simulink model "SMR_1MW_model"  (R2025b)
settings: Solver=daessc  StartTime=0.0  StopTime=60*80  RelTol=1e-3
libraries: fl_lib x41, nesl_utility x29, RankineCycle_lib x3, simulink x2, slpidlib x2
(part 2 of 2)

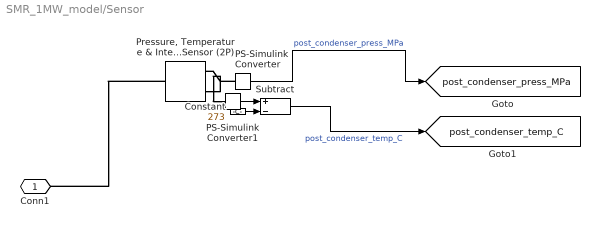
== system SMR_1MW_model/Sensor ==
  Constant : Constant  Value=273
  PS-Simulink Converter : nesl_utility/PS-Simulink Converter  PhysicalDomain=network_engine_domain  SubClassName=ps_output  LeftPortType=input  RightPortType=output  PseudoPeriodic=off  Frequencies=[]  VectorFormat=inherit  Unit=inherit  AffineConversion=off
  PS-Simulink Converter1 : nesl_utility/PS-Simulink Converter  PhysicalDomain=network_engine_domain  SubClassName=ps_output  LeftPortType=input  RightPortType=output  PseudoPeriodic=off  Frequencies=[]  VectorFormat=inherit  Unit=inherit  AffineConversion=off
  "Pressure, Temperature & Internal Energy Sensor (2P)" : fl_lib/Two-Phase Fluid/Sensors/Pressure, Temperature & Internal Energy Sensor (2P)  reference=foundation.enum.MeasurementReference.absolute  pressure=true  pressure_spec=foundation.enum.PressureMeasementSpec.Absolute  temperature=true  internal_energy=false
      settings: InternalSimscapePortConfiguration="{\"Bottom\":[{\"id\":\"T\",\"label\":\"T\",\"type\":\"output\"}],\"Left\":[{\"id\":\"A\",\"label\":\"A\",\"type\":\"foundation.two_phase_fluid.two_phase_fluid\"}],\"Right\":[{\"id\":\"Pa\",\"label\":\"Pa\",\"type\":\"output\"}],\"Top\":[]}"
  Subtract : Sum  Inputs=+-
  Conn1 : PMIOPort  Side=Left
  tag scope: post_condenser_press_MPa=global, post_condenser_temp_C=global
  wires:
  PS-Simulink Converter/1 -> [post_condenser_press_MPa]  "post_condenser_press_MPa"
  PS-Simulink Converter1/1 -> Subtract/1
  Constant/1 -> Subtract/2
  Subtract/1 -> [post_condenser_temp_C]  "post_condenser_temp_C"
  connections:
  PS-Simulink Converter/LConn1 -- "Pressure, Temperature & Internal Energy Sensor (2P)"/RConn1
  "Pressure, Temperature & Internal Energy Sensor (2P)"/RConn2 -- PS-Simulink Converter1/LConn1
  "Pressure, Temperature & Internal Energy Sensor (2P)"/LConn1 -- Conn1/RConn1

== system SMR_1MW_model/Sensors ==
  Subsystem4 : Subsystem
  Conn1 : PMIOPort  Side=Right
  tag scope: pre_trubine_temp_C=global, pre_turbine_press_MPa=global
  wires:
  Subsystem4/1(pressure) -> [pre_turbine_press_MPa]  "pre-turbine_press_MPa"
  Subsystem4/2(temperature) -> [pre_trubine_temp_C]  "pre-trubine_temp_C"
  connections:
  Subsystem4/LConn1 -- Conn1/RConn1

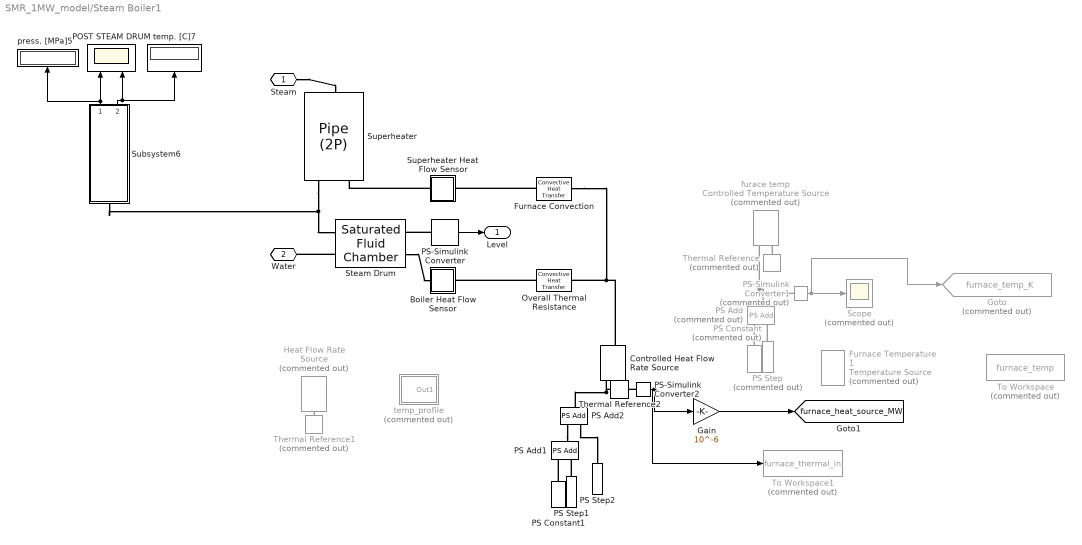
== system SMR_1MW_model/Steam Boiler1 ==
  Boiler Heat Flow Sensor : Subsystem
  Controlled Heat Flow Rate Source : fl_lib/Thermal/Thermal Sources/Controlled Heat Flow Rate Source
  Furnace Convection : fl_lib/Thermal/Thermal Elements/Convective Heat Transfer  thermal_type=foundation.enum.constant_variable.constant  area=pi * sqrt(4*0.01/pi) * 4+ 2 m^2  heat_tr_coeff=heater_heat_coeff W/(m^2 * K)  min_heat_tr_coeff=1e-3 W/(K*m^2)  T_specify=off  T_priority=None  T=0 K  T_nominal_specify=off  T_nominal_value=1  T_nominal_unit=K  Q_specify=off  Q_priority=None  Q=0 W  Q_nominal_specify=off  Q_nominal_value=1  Q_nominal_unit=W
  Furnace Temperature1 : fl_lib/Thermal/Thermal Sources/Temperature Source  Commented=on  temperature=T_furnace degC
  Gain : Gain  Gain=10^-6
  Goto : Goto  Commented=on  GotoTag=furnace_temp_K  TagVisibility=global
  Heat Flow Rate Source : fl_lib/Thermal/Thermal Sources/Heat Flow Rate Source  Commented=on  heat_flow=core_thermal_MW MW
      settings: InternalSimscapePortConfiguration="{\"Bottom\":[],\"Left\":[{\"id\":\"B\",\"label\":\"B\",\"type\":\"foundation.thermal.thermal\"}],\"Right\":[{\"id\":\"A\",\"label\":\"A\",\"type\":\"foundation.thermal.thermal\"}],\"Top\":[]}"
  Overall Thermal Resistance : fl_lib/Thermal/Thermal Elements/Convective Heat Transfer  thermal_type=foundation.enum.constant_variable.constant  area=boiler_area m^2  heat_tr_coeff=heater_heat_coeff W/(m^2 * K)  min_heat_tr_coeff=1e-3 W/(K*m^2)  T_specify=off  T_priority=None  T=0 K  T_nominal_specify=off  T_nominal_value=1  T_nominal_unit=K  Q_specify=off  Q_priority=None  Q=0 W  Q_nominal_specify=off  Q_nominal_value=1  Q_nominal_unit=W
  POST STEAM DRUM : Scope  NumInputPorts=2
      settings: ActiveDisplayYMinimum=0.96271  ActiveDisplayYMaximum=1.5597  DataLoggingVariableName=ScopeData3
  PS Add : fl_lib/Physical Signals/Functions/PS Add  Commented=on
  PS Add1 : fl_lib/Physical Signals/Functions/PS Add
  PS Add2 : fl_lib/Physical Signals/Functions/PS Add
  PS Constant : fl_lib/Physical Signals/Sources/PS Constant  Commented=on  constant=T_furnace+273
  PS Constant1 : fl_lib/Physical Signals/Sources/PS Constant  constant=core_thermal_MW*10^6
  PS Step : fl_lib/Physical Signals/Sources/PS Step  Commented=on  step_time=60*40 s  initial_value=0  final_value=temp_step
  PS Step1 : fl_lib/Physical Signals/Sources/PS Step  step_time=60*40 s  initial_value=0  final_value=thermal_step*10^6
  PS Step2 : fl_lib/Physical Signals/Sources/PS Step  step_time=60*60 s  initial_value=0  final_value=-thermal_step*10^6
  PS-Simulink Converter : nesl_utility/PS-Simulink Converter  PhysicalDomain=network_engine_domain  SubClassName=ps_output  LeftPortType=input  RightPortType=output  PseudoPeriodic=off  Frequencies=[]  VectorFormat=1-D array  Unit=1  AffineConversion=off
  PS-Simulink Converter1 : nesl_utility/PS-Simulink Converter  Commented=on  PhysicalDomain=network_engine_domain  SubClassName=ps_output  LeftPortType=input  RightPortType=output  PseudoPeriodic=off  Frequencies=[]  VectorFormat=inherit  Unit=inherit  AffineConversion=off
  PS-Simulink Converter2 : nesl_utility/PS-Simulink Converter  PhysicalDomain=network_engine_domain  SubClassName=ps_output  LeftPortType=input  RightPortType=output  PseudoPeriodic=off  Frequencies=[]  VectorFormat=inherit  Unit=inherit  AffineConversion=off
  Scope : Scope  Commented=on
      settings: ActiveDisplayYMinimum=-1  ActiveDisplayYMaximum=1  DataLoggingVariableName=ScopeData2
  Steam Drum : RankineCycle_lib/Saturated Fluid Chamber  volume=boiler_volume m^3  area_A=0.01 m^2  area_B=0.01 m^2  L_min=0.01  L_max=0.99  p_I_specify=on  p_I_priority=High  p_I=p_init MPa  p_I_nominal_specify=off  p_I_nominal_value=1  p_I_nominal_unit=MPa  L_specify=on  L_priority=High  L=L_init  L_nominal_specify=off  L_nominal_value=1  L_nominal_unit=1
      settings: InternalSimscapePortConfiguration="{\"Bottom\":[],\"Left\":[{\"id\":\"A\",\"label\":\"A\",\"type\":\"foundation.two_phase_fluid.two_phase_fluid\"},{\"id\":\"B\",\"label\":\"B\",\"type\":\"foundation.two_phase_fluid.two_phase_fluid\"}],\"Right\":[{\"id\":\"L_out\",\"label\":\"L\",\"type\":\"output\"},{\"id\":\"H\",\"label\":\"H\",\"type\":\"foundation.thermal.thermal\"}],\"Top\":[]}"
  Subsystem6 : Subsystem
  Superheater : fl_lib/Two-Phase Fluid/Elements/Pipe (2P)  length=4 m  area=0.01 m^2  Dh=sqrt(4*0.01/pi) m  length_add=0.1 * 4 m  roughness=15e-6 m  Re_lam=2000  Re_tur=4000  shape_factor=64  Nu_lam=3.66  inertia=true  energy_spec=foundation.enum.energy_spec.temperature  p_init=p_init MPa  T_init=T_init degC  x_init=0.2  alpha_init=0.5  h_init=1500 kJ/kg  u_init=1500 kJ/kg  mdot_init=0 kg/s  time_constant=0.1 s
      settings: InternalSimscapePortConfiguration="{\"Bottom\":[],\"Left\":[{\"id\":\"A\",\"label\":\"A\",\"type\":\"foundation.two_phase_fluid.two_phase_fluid\"},{\"id\":\"H\",\"label\":\"H\",\"type\":\"foundation.thermal.thermal\"}],\"Right\":[{\"id\":\"B\",\"label\":\"B\",\"type\":\"foundation.two_phase_fluid.two_phase_fluid\"}],\"Top\":[]}"
  Superheater Heat Flow Sensor : Subsystem
  Thermal Reference : fl_lib/Thermal/Thermal Elements/Thermal Reference  Commented=on
  Thermal Reference1 : fl_lib/Thermal/Thermal Elements/Thermal Reference  Commented=on
  Thermal Reference2 : fl_lib/Thermal/Thermal Elements/Thermal Reference
  To Workspace : ToWorkspace  Commented=on  VariableName=furnace_temp  SaveFormat=Timeseries  SampleTime=0.5
  To Workspace1 : ToWorkspace  Commented=on  VariableName=furnace_thermal_in  SaveFormat=Structure With Time  SampleTime=0.5
  furace temp : fl_lib/Thermal/Thermal Sources/Controlled Temperature Source  Commented=on
  press. [MPa]5 : Display
  temp. [C]7 : Display
  temp_profile : Subsystem  Commented=on
      settings: PortSchema="{\"entries\":[{\"content\":{\"sides\":[{\"content\":{},\"type\":\"ConnectorPlacement.EquallySpacedRectSide\",\"uuid\":\"68a2c157-fc1f-4d74-a1de-170950004e54\"},{\"content\":{\"connectorIds\":[\"Out1\"],\"side\":\"RIGHT\"},\"type\":\"ConnectorPlacement.EquallySpacedRectSide\",\"uuid\":\"f36b84c4-e68c-441f-b2e1-01bcb91045b0\"},{\"content\":{\"connectorIds\":[\"LConn1\"],\"side\":\"TOP\"},\"type\":\"ConnectorPlacement.EquallySpacedRectSide\",\"uuid\":\"323f1c28-fa68-49ae-bcd7-539ae4c64026\"}]},\"type\":\"ConnectorPlacement.EquallySpacedConnector\",\"uuid\":\"ae9f05fe-dbd5-4844-ab6c-bbb2ab4d97c5\"}],\"packageUris\":[\"http://schema.mathworks.com/mf0/Connector/R2020b\"],\"version\":\"1.0\"}"
  Steam : PMIOPort  Side=Left
  Water : PMIOPort  Port=2  Side=Left
  Level : Outport  VectorParamsAs1DForOutWhenUnconnected=off
  tag scope: furnace_heat_source_MW=global
  wires:
  PS-Simulink Converter/1 -> Level/1
  PS-Simulink Converter1/1 -> Goto/1, Scope/1
  Subsystem6/2(temperature) -> temp. [C]7/1, POST STEAM DRUM/2
  Subsystem6/1(pressure) -> press. [MPa]5/1, POST STEAM DRUM/1
  ? -> To Workspace/1
  PS-Simulink Converter2/1 -> To Workspace1/1, Gain/1
  Gain/1 -> [furnace_heat_source_MW]
  connections:
  Steam Drum/LConn2 -- Water/RConn1
  PS-Simulink Converter/LConn1 -- Steam Drum/RConn1
  Furnace Convection/LConn1 -- Overall Thermal Resistance/LConn1 -- Controlled Heat Flow Rate Source/LConn1
  Overall Thermal Resistance/RConn1 -- Boiler Heat Flow Sensor/LConn1
  Furnace Convection/RConn1 -- Superheater Heat Flow Sensor/LConn1
  Steam Drum/RConn2 -- Boiler Heat Flow Sensor/RConn1
  Superheater Heat Flow Sensor/RConn1 -- Superheater/LConn2
  Steam/RConn1 -- Superheater/RConn1
  Superheater/LConn1 -- Subsystem6/LConn1 -- Steam Drum/LConn1
  Thermal Reference/LConn1 -- furace temp/RConn2
  Thermal Reference1/LConn1 -- Heat Flow Rate Source/RConn1
  PS Constant/RConn1 -- PS Add/LConn1
  PS Step/RConn1 -- PS Add/LConn2
  PS Add/RConn1 -- furace temp/RConn1 -- PS-Simulink Converter1/LConn1
  PS Step1/RConn1 -- PS Add1/LConn2
  PS Constant1/RConn1 -- PS Add1/LConn1
  Thermal Reference2/LConn1 -- Controlled Heat Flow Rate Source/RConn2
  PS Add2/LConn1 -- PS Add1/RConn1
  PS Add2/RConn1 -- PS-Simulink Converter2/LConn1 -- Controlled Heat Flow Rate Source/RConn1
  PS Add2/LConn2 -- PS Step2/RConn1

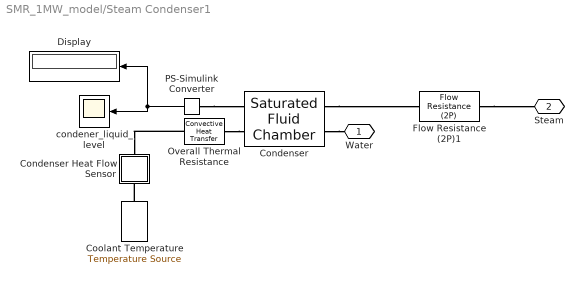
== system SMR_1MW_model/Steam Condenser1 ==
  Condenser : RankineCycle_lib/Saturated Fluid Chamber  volume=8 m^3  area_A=0.05 m^2  area_B=0.05 m^2  L_min=0.01  L_max=0.99  p_I_specify=on  p_I_priority=High  p_I=10 kPa  p_I_nominal_specify=off  p_I_nominal_value=1  p_I_nominal_unit=MPa  L_specify=on  L_priority=High  L=0.5  L_nominal_specify=off  L_nominal_value=1  L_nominal_unit=1
      settings: InternalSimscapePortConfiguration="{\"Bottom\":[],\"Left\":[{\"id\":\"A\",\"label\":\"A\",\"type\":\"foundation.two_phase_fluid.two_phase_fluid\"},{\"id\":\"B\",\"label\":\"B\",\"type\":\"foundation.two_phase_fluid.two_phase_fluid\"}],\"Right\":[{\"id\":\"L_out\",\"label\":\"L\",\"type\":\"output\"},{\"id\":\"H\",\"label\":\"H\",\"type\":\"foundation.thermal.thermal\"}],\"Top\":[]}"
  Condenser Heat Flow Sensor : Subsystem
  Coolant Temperature : fl_lib/Thermal/Thermal Sources/Temperature Source  temperature=2 degC
  Display : Display
  Flow Resistance (2P)1 : fl_lib/Two-Phase Fluid/Elements/Flow Resistance (2P)  delta_p_nominal=0.001 MPa  mdot_nominal=1.5 kg/s  v_nominal=0 m^3/kg  area=0.02 m^2  laminar_fraction=1e-3
      settings: InternalSimscapePortConfiguration="{\"Bottom\":[],\"Left\":[{\"id\":\"A\",\"label\":\"A\",\"type\":\"foundation.two_phase_fluid.two_phase_fluid\"}],\"Right\":[{\"id\":\"B\",\"label\":\"B\",\"type\":\"foundation.two_phase_fluid.two_phase_fluid\"}],\"Top\":[]}"
  Overall Thermal Resistance : fl_lib/Thermal/Thermal Elements/Convective Heat Transfer  thermal_type=foundation.enum.constant_variable.constant  area=20 m^2  heat_tr_coeff=4000 W/(m^2 * K)  min_heat_tr_coeff=1e-3 W/(K*m^2)  T_specify=off  T_priority=None  T=0 K  T_nominal_specify=off  T_nominal_value=1  T_nominal_unit=K  Q_specify=off  Q_priority=None  Q=0 W  Q_nominal_specify=off  Q_nominal_value=1  Q_nominal_unit=W
  PS-Simulink Converter : nesl_utility/PS-Simulink Converter  PhysicalDomain=network_engine_domain  SubClassName=ps_output  LeftPortType=input  RightPortType=output  PseudoPeriodic=off  Frequencies=[]  VectorFormat=inherit  Unit=inherit  AffineConversion=off
  condener_liquid_level : Scope
      settings: ActiveDisplayYMinimum=0.22633  ActiveDisplayYMaximum=0.53308  DataLoggingVariableName=ScopeData3
  Water : PMIOPort  Side=Left
  Steam : PMIOPort  Port=2  Side=Right
  wires:
  PS-Simulink Converter/1 -> Display/1, condener_liquid_level/1
  connections:
  Overall Thermal Resistance/RConn1 -- Condenser/RConn2
  Condenser/LConn2 -- Water/RConn1
  Coolant Temperature/LConn1 -- Condenser Heat Flow Sensor/RConn1
  Overall Thermal Resistance/LConn1 -- Condenser Heat Flow Sensor/LConn1
  Flow Resistance (2P)1/LConn1 -- Steam/RConn1
  PS-Simulink Converter/LConn1 -- Condenser/RConn1
  Condenser/LConn1 -- Flow Resistance (2P)1/RConn1

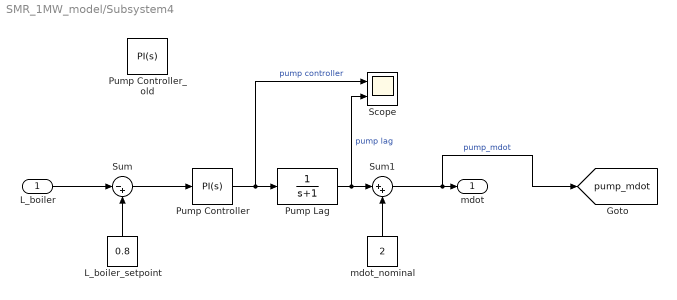
== system SMR_1MW_model/Subsystem4 ==
  L_boiler : Inport
  L_boiler_setpoint : Constant  Value=0.8
  Pump Controller : slpidlib/PID Controller  Controller=PI  Form=Ideal  TimeDomain=Continuous-time  UseExternalTs=off  SampleTime=-1  IntegratorMethod=Forward Euler  FilterMethod=Forward Euler  ControllerParametersSource=internal  P=313.074531987638  I=0.0123881397923726  UseKiTs=off  D=3.11324990368256  UseExternalDerivativeSource=off  N=0.464746256313806  UseFilter=on  TunerSelectOption=Transfer Function Based (PID Tuner App)  InitialConditionSource=internal  InitialConditionForIntegrator=0.1  InitialConditionForFilter=0  DifferentiatorICPrevScaledInput=0  ExternalReset=none  TrackingMode=off  Kt=1  LimitOutput=on  SatLimitsSource=internal  UpperSaturationLimit=5  LowerSaturationLimit=-1.5  LinearizeAsGain=on  AntiWindupMode=back-calculation  Kb=1  LimitIntegrator=off  UpperIntegratorSaturationLimit=inf  LowerIntegratorSaturationLimit=-inf  POutMin=[]  POutMax=[]  IOutMin=[]  IOutMax=[]  DOutMin=[]  DOutMax=[]  NOutMin=[]  NOutMax=[]  SumOutMin=[]  SumOutMax=[]  SaturationOutMin=[]  SaturationOutMax=[]  PParamMin=[]  PParamMax=[]  IParamMin=[]  IParamMax=[]  DParamMin=[]  DParamMax=[]  NParamMin=[]  NParamMax=[]  KbParamMin=[]  KbParamMax=[]  KtParamMin=[]  KtParamMax=[]  KbOutMin=[]  KbOutMax=[]  KtOutMin=[]  KtOutMax=[]  IntegratorOutMin=[]  IntegratorOutMax=[]  FilterOutMin=[]  FilterOutMax=[]  SumI1OutMin=[]  SumI1OutMax=[]  SumI2OutMin=[]  SumI2OutMax=[]  SumI3OutMin=[]  SumI3OutMax=[]  SumI4OutMin=[]  SumI4OutMax=[]  SumDOutMin=[]  SumDOutMax=[]  DifferentiatorOutMin=[]  DifferentiatorOutMax=[]  FilterDiffOutCoefMin=[]  FilterDiffOutCoefMax=[]  ReciprocalOutMin=[]  ReciprocalOutMax=[]  SumDenOutMin=[]  SumDenOutMax=[]  SumNumOutMin=[]  SumNumOutMax=[]  DivideOutMin=[]  DivideOutMax=[]  UdiffTsProdOutMin=[]  UdiffTsProdOutMax=[]  NTsProdOutMin=[]  NTsProdOutMax=[]  UintegralTsProdOutMin=[]  UintegralTsProdOutMax=[]  UngainTsProdOutMin=[]  UngainTsProdOutMax=[]  ClampingZeroOutDataTypeStr=Inherit: Inherit via back propagation  ClampingZeroOutMin=[]  ClampingZeroOutMax=[]  FilterDenConstantOutDataTypeStr=Inherit: Inherit via back propagation  FilterDenConstantOutMin=[]  FilterDenConstantOutMax=[]  PCopyOutDataTypeStr=Inherit: Inherit via back propagation  PCopyOutMin=[]  PCopyOutMax=[]  NCopyOutDataTypeStr=Inherit: Inherit via back propagation  NCopyOutMin=[]  NCopyOutMax=[]  IntegratorContinuousStateAttributes=''  IntegratorStateMustResolveToSignalObject=off  IntegratorRTWStateStorageClass=Auto  FilterContinuousStateAttributes=''  FilterStateMustResolveToSignalObject=off  FilterRTWStateStorageClass=Auto  ParallelPVariant=Passthrough  IdealPVariant=InternalParameters  IVariant=InternalParameters  DVariant=Disabled  IntegratorVariant=Continuous  SatVariant=Enabled  AWVariant=BackCalculation  PCopyVariant=Disabled  TRVariant=Disabled  FdbkBlocksVariant=Forward  IdealPFdbkVariant=Disabled  SatFdbkVariant=Disabled  DerivativeFilterVariant=Disabled  NVariant=Disabled  NCopyVariant=Disabled_SignalSpec  FilterICVariant=Disabled  IntegratorICVariant=InternalICs  ExternalResetVariant=Disabled  TRSumVariant=Passthrough  SumFdbkVariant=Disabled  SumVariant=Sum_PI  TsampFilterVariant=InternalTs  TsampNgainVariant=Passthrough  TsampIntegralVariant=Disabled_SignalSpec  ExternalSaturationOutDataTypeStr=Inherit: Same as second input  DerivativeSourceVariant=Disabled  PreIntVariant=InternalPreInt
  Pump Controller_old : slpidlib/PID Controller  Controller=PI  Form=Ideal  TimeDomain=Continuous-time  UseExternalTs=off  SampleTime=-1  IntegratorMethod=Forward Euler  FilterMethod=Forward Euler  ControllerParametersSource=internal  P=313.074531987638  I=0.0123881397923726  UseKiTs=off  D=3.11324990368256  UseExternalDerivativeSource=off  N=0.464746256313806  UseFilter=on  TunerSelectOption=Transfer Function Based (PID Tuner App)  InitialConditionSource=internal  InitialConditionForIntegrator=0.1  InitialConditionForFilter=0  DifferentiatorICPrevScaledInput=0  ExternalReset=none  TrackingMode=off  Kt=1  LimitOutput=on  SatLimitsSource=internal  UpperSaturationLimit=5  LowerSaturationLimit=-1.5  LinearizeAsGain=on  AntiWindupMode=back-calculation  Kb=1  LimitIntegrator=off  UpperIntegratorSaturationLimit=inf  LowerIntegratorSaturationLimit=-inf  POutMin=[]  POutMax=[]  IOutMin=[]  IOutMax=[]  DOutMin=[]  DOutMax=[]  NOutMin=[]  NOutMax=[]  SumOutMin=[]  SumOutMax=[]  SaturationOutMin=[]  SaturationOutMax=[]  PParamMin=[]  PParamMax=[]  IParamMin=[]  IParamMax=[]  DParamMin=[]  DParamMax=[]  NParamMin=[]  NParamMax=[]  KbParamMin=[]  KbParamMax=[]  KtParamMin=[]  KtParamMax=[]  KbOutMin=[]  KbOutMax=[]  KtOutMin=[]  KtOutMax=[]  IntegratorOutMin=[]  IntegratorOutMax=[]  FilterOutMin=[]  FilterOutMax=[]  SumI1OutMin=[]  SumI1OutMax=[]  SumI2OutMin=[]  SumI2OutMax=[]  SumI3OutMin=[]  SumI3OutMax=[]  SumI4OutMin=[]  SumI4OutMax=[]  SumDOutMin=[]  SumDOutMax=[]  DifferentiatorOutMin=[]  DifferentiatorOutMax=[]  FilterDiffOutCoefMin=[]  FilterDiffOutCoefMax=[]  ReciprocalOutMin=[]  ReciprocalOutMax=[]  SumDenOutMin=[]  SumDenOutMax=[]  SumNumOutMin=[]  SumNumOutMax=[]  DivideOutMin=[]  DivideOutMax=[]  UdiffTsProdOutMin=[]  UdiffTsProdOutMax=[]  NTsProdOutMin=[]  NTsProdOutMax=[]  UintegralTsProdOutMin=[]  UintegralTsProdOutMax=[]  UngainTsProdOutMin=[]  UngainTsProdOutMax=[]  ClampingZeroOutDataTypeStr=Inherit: Inherit via back propagation  ClampingZeroOutMin=[]  ClampingZeroOutMax=[]  FilterDenConstantOutDataTypeStr=Inherit: Inherit via back propagation  FilterDenConstantOutMin=[]  FilterDenConstantOutMax=[]  PCopyOutDataTypeStr=Inherit: Inherit via back propagation  PCopyOutMin=[]  PCopyOutMax=[]  NCopyOutDataTypeStr=Inherit: Inherit via back propagation  NCopyOutMin=[]  NCopyOutMax=[]  IntegratorContinuousStateAttributes=''  IntegratorStateMustResolveToSignalObject=off  IntegratorRTWStateStorageClass=Auto  FilterContinuousStateAttributes=''  FilterStateMustResolveToSignalObject=off  FilterRTWStateStorageClass=Auto  ParallelPVariant=Passthrough  IdealPVariant=InternalParameters  IVariant=InternalParameters  DVariant=Disabled  IntegratorVariant=Continuous  SatVariant=Enabled  AWVariant=BackCalculation  PCopyVariant=Disabled  TRVariant=Disabled  FdbkBlocksVariant=Forward  IdealPFdbkVariant=Disabled  SatFdbkVariant=Disabled  DerivativeFilterVariant=Disabled  NVariant=Disabled  NCopyVariant=Disabled_SignalSpec  FilterICVariant=Disabled  IntegratorICVariant=InternalICs  ExternalResetVariant=Disabled  TRSumVariant=Passthrough  SumFdbkVariant=Disabled  SumVariant=Sum_PI  TsampFilterVariant=InternalTs  TsampNgainVariant=Passthrough  TsampIntegralVariant=Disabled_SignalSpec  ExternalSaturationOutDataTypeStr=Inherit: Same as second input  DerivativeSourceVariant=Disabled  PreIntVariant=InternalPreInt
  Pump Lag : TransferFcn  Denominator=[1 1]
  Scope : Scope  NumInputPorts=2
      settings: ActiveDisplayYMinimum=-362.81394  ActiveDisplayYMaximum=174.22132  DataLoggingVariableName=ScopeData2
  Sum : Sum  Inputs=|-+
  Sum1 : Sum  Inputs=|++
  mdot_nominal : Constant  Value=2
  mdot : Outport  VectorParamsAs1DForOutWhenUnconnected=off
  tag scope: pump_mdot=global
  wires:
  L_boiler_setpoint/1 -> Sum/2
  Sum1/1 -> [pump_mdot], mdot/1  "pump_mdot"
  Pump Controller/1 -> Scope/1, Pump Lag/1  "pump controller"
  mdot_nominal/1 -> Sum1/2
  Pump Lag/1 -> Scope/2, Sum1/1  "pump lag"
  L_boiler/1 -> Sum/1
  Sum/1 -> Pump Controller/1

== system SMR_1MW_model/enthalpy ==
  PS-Simulink Converter : nesl_utility/PS-Simulink Converter  PhysicalDomain=network_engine_domain  SubClassName=ps_output  LeftPortType=input  RightPortType=output  PseudoPeriodic=off  Frequencies=[]  VectorFormat=inherit  Unit=inherit  AffineConversion=off
  Scope2 : Scope
      settings: ActiveDisplayYMinimum=3240.8629202811012  ActiveDisplayYMaximum=3406.8144304703646  DataLoggingVariableName=ScopeData8
  Thermodynamic Properties Sensor (2P) : fl_lib/Two-Phase Fluid/Sensors/Thermodynamic Properties Sensor (2P)  temperature=false  enthalpy=true  density=false  specific_volume=false  entropy=false
      settings: InternalSimscapePortConfiguration="{\"Bottom\":[],\"Left\":[{\"id\":\"A\",\"label\":\"A\",\"type\":\"foundation.two_phase_fluid.two_phase_fluid\"}],\"Right\":[{\"id\":\"H\",\"label\":\"h\",\"type\":\"output\"}],\"Top\":[]}"
  Conn1 : PMIOPort  Side=Left
  tag scope: enthalpy=global
  wires:
  PS-Simulink Converter/1 -> [enthalpy], Scope2/1
  connections:
  PS-Simulink Converter/LConn1 -- Thermodynamic Properties Sensor (2P)/RConn1
  Thermodynamic Properties Sensor (2P)/LConn1 -- Conn1/RConn1

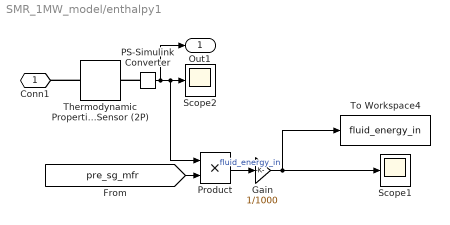
== system SMR_1MW_model/enthalpy1 ==
  Gain : Gain  Gain=1/1000
  PS-Simulink Converter : nesl_utility/PS-Simulink Converter  PhysicalDomain=network_engine_domain  SubClassName=ps_output  LeftPortType=input  RightPortType=output  PseudoPeriodic=off  Frequencies=[]  VectorFormat=inherit  Unit=inherit  AffineConversion=off
  Product : Product
  Scope1 : Scope
      settings: ActiveDisplayYMinimum=0.070137777487190744  ActiveDisplayYMaximum=0.32891510701589166  DataLoggingVariableName=ScopeData13
  Scope2 : Scope
      settings: ActiveDisplayYMinimum=146.80010359013045  ActiveDisplayYMaximum=197.88345173033352  DataLoggingVariableName=ScopeData8
  Thermodynamic Properties Sensor (2P) : fl_lib/Two-Phase Fluid/Sensors/Thermodynamic Properties Sensor (2P)  temperature=false  enthalpy=true  density=false  specific_volume=false  entropy=false
      settings: InternalSimscapePortConfiguration="{\"Bottom\":[],\"Left\":[{\"id\":\"A\",\"label\":\"A\",\"type\":\"foundation.two_phase_fluid.two_phase_fluid\"}],\"Right\":[{\"id\":\"H\",\"label\":\"h\",\"type\":\"output\"}],\"Top\":[]}"
  To Workspace4 : ToWorkspace  VariableName=fluid_energy_in  SaveFormat=Structure With Time  SampleTime=0.5
  Conn1 : PMIOPort  Side=Left
  Out1 : Outport
  wires:
  PS-Simulink Converter/1 -> Out1/1, Product/1, Scope2/1
  [pre_sg_mfr] -> Product/2
  Product/1 -> Gain/1  "fluid_energy_in"
  Gain/1 -> To Workspace4/1, Scope1/1
  connections:
  PS-Simulink Converter/LConn1 -- Thermodynamic Properties Sensor (2P)/RConn1
  Thermodynamic Properties Sensor (2P)/LConn1 -- Conn1/RConn1

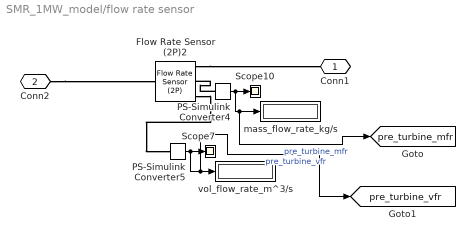
== system SMR_1MW_model/flow rate sensor ==
  Flow Rate Sensor (2P)2 : fl_lib/Two-Phase Fluid/Sensors/Flow Rate Sensor (2P)  mass_flow_measure=true  volumetric_flow_measure=true  energy_flow_measure=false
      settings: InternalSimscapePortConfiguration="{\"Bottom\":[],\"Left\":[{\"id\":\"A\",\"label\":\"A\",\"type\":\"foundation.two_phase_fluid.two_phase_fluid\"}],\"Right\":[{\"id\":\"B\",\"label\":\"B\",\"type\":\"foundation.two_phase_fluid.two_phase_fluid\"},{\"id\":\"M\",\"label\":\"M\",\"type\":\"output\"},{\"id\":\"V\",\"label\":\"V\",\"type\":\"output\"}],\"Top\":[]}"
  PS-Simulink Converter4 : nesl_utility/PS-Simulink Converter  PhysicalDomain=network_engine_domain  SubClassName=ps_output  LeftPortType=input  RightPortType=output  PseudoPeriodic=off  Frequencies=[]  VectorFormat=inherit  Unit=inherit  AffineConversion=off
  PS-Simulink Converter5 : nesl_utility/PS-Simulink Converter  PhysicalDomain=network_engine_domain  SubClassName=ps_output  LeftPortType=input  RightPortType=output  PseudoPeriodic=off  Frequencies=[]  VectorFormat=inherit  Unit=inherit  AffineConversion=off
  Scope10 : Scope
      settings: ActiveDisplayYMinimum=1.1711652570922302  ActiveDisplayYMaximum=1.2205215489129049
  Scope7 : Scope
      settings: ActiveDisplayYMinimum=0.24234  ActiveDisplayYMaximum=0.24528  DataLoggingVariableName=ScopeData6
  mass_flow_rate_kg/s : Display
  vol_flow_rate_m^3/s : Display
  Conn1 : PMIOPort  Side=Right
  Conn2 : PMIOPort  Port=2  Side=Left
  tag scope: pre_turbine_mfr=global, pre_turbine_vfr=global
  wires:
  PS-Simulink Converter5/1 -> [pre_turbine_vfr], vol_flow_rate_m^3/s/1, Scope7/1  "pre_turbine_vfr"
  PS-Simulink Converter4/1 -> [pre_turbine_mfr], mass_flow_rate_kg/s/1, Scope10/1  "pre_turbine_mfr"
  connections:
  PS-Simulink Converter4/LConn1 -- Flow Rate Sensor (2P)2/RConn2
  Flow Rate Sensor (2P)2/RConn1 -- Conn1/RConn1
  Flow Rate Sensor (2P)2/RConn3 -- PS-Simulink Converter5/LConn1
  Conn2/RConn1 -- Flow Rate Sensor (2P)2/LConn1

== system SMR_1MW_model/flow rate sensor 1 ==
  Flow Rate Sensor (2P)3 : fl_lib/Two-Phase Fluid/Sensors/Flow Rate Sensor (2P)  mass_flow_measure=true  volumetric_flow_measure=false  energy_flow_measure=false
      settings: InternalSimscapePortConfiguration="{\"Bottom\":[],\"Left\":[{\"id\":\"A\",\"label\":\"A\",\"type\":\"foundation.two_phase_fluid.two_phase_fluid\"}],\"Right\":[{\"id\":\"B\",\"label\":\"B\",\"type\":\"foundation.two_phase_fluid.two_phase_fluid\"},{\"id\":\"M\",\"label\":\"M\",\"type\":\"output\"}],\"Top\":[]}"
  PS-Simulink Converter3 : nesl_utility/PS-Simulink Converter  PhysicalDomain=network_engine_domain  SubClassName=ps_output  LeftPortType=input  RightPortType=output  PseudoPeriodic=off  Frequencies=[]  VectorFormat=inherit  Unit=inherit  AffineConversion=off
  Scope15 : Scope
      settings: ActiveDisplayYMinimum=-1.91068  ActiveDisplayYMaximum=0.2134  DataLoggingVariableName=ScopeData5
  mass_flow_rate : Display
  Conn1 : PMIOPort  Side=Right
  Conn2 : PMIOPort  Port=2  Side=Left
  tag scope: pre_sg_mfr=global
  wires:
  PS-Simulink Converter3/1 -> [pre_sg_mfr], Scope15/1, mass_flow_rate/1  "pre_sg_mfr"
  connections:
  PS-Simulink Converter3/LConn1 -- Flow Rate Sensor (2P)3/RConn2
  Flow Rate Sensor (2P)3/LConn1 -- Conn2/RConn1
  Flow Rate Sensor (2P)3/RConn1 -- Conn1/RConn1

== system SMR_1MW_model/flow rate sensor 2 ==
  Flow Rate Sensor (2P)3 : fl_lib/Two-Phase Fluid/Sensors/Flow Rate Sensor (2P)  mass_flow_measure=false  volumetric_flow_measure=true  energy_flow_measure=false
      settings: InternalSimscapePortConfiguration="{\"Bottom\":[],\"Left\":[{\"id\":\"A\",\"label\":\"A\",\"type\":\"foundation.two_phase_fluid.two_phase_fluid\"}],\"Right\":[{\"id\":\"B\",\"label\":\"B\",\"type\":\"foundation.two_phase_fluid.two_phase_fluid\"},{\"id\":\"V\",\"label\":\"V\",\"type\":\"output\"}],\"Top\":[]}"
  PS-Simulink Converter3 : nesl_utility/PS-Simulink Converter  PhysicalDomain=network_engine_domain  SubClassName=ps_output  LeftPortType=input  RightPortType=output  PseudoPeriodic=off  Frequencies=[]  VectorFormat=inherit  Unit=inherit  AffineConversion=off
  Scope15 : Scope
      settings: ActiveDisplayYMinimum=-1.91068  ActiveDisplayYMaximum=0.2134  DataLoggingVariableName=ScopeData5
  vol_flow_rate1 : Display
  Conn1 : PMIOPort  Side=Right
  Conn2 : PMIOPort  Port=2  Side=Left
  tag scope: post_condenser_vfr=global
  wires:
  PS-Simulink Converter3/1 -> [post_condenser_vfr], Scope15/1, vol_flow_rate1/1  "post_condenser_vfr"
  connections:
  PS-Simulink Converter3/LConn1 -- Flow Rate Sensor (2P)3/RConn2
  Flow Rate Sensor (2P)3/LConn1 -- Conn2/RConn1
  Flow Rate Sensor (2P)3/RConn1 -- Conn1/RConn1

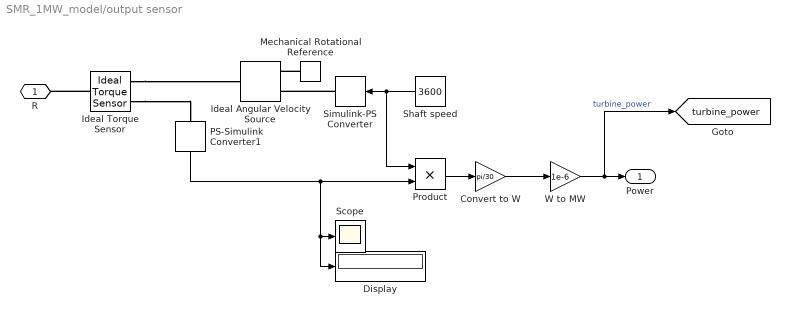
== system SMR_1MW_model/output sensor ==
  Convert to W : Gain  Gain=pi/30
  Display : Display
  Ideal Angular Velocity Source : fl_lib/Mechanical/Mechanical Sources/Ideal Angular Velocity Source
  Ideal Torque Sensor : fl_lib/Mechanical/Mechanical Sensors/Ideal Torque Sensor
  Mechanical Rotational Reference : fl_lib/Mechanical/Rotational Elements/Mechanical Rotational Reference
  PS-Simulink Converter1 : nesl_utility/PS-Simulink Converter  PhysicalDomain=network_engine_domain  SubClassName=ps_output  LeftPortType=input  RightPortType=output  PseudoPeriodic=off  Frequencies=[]  VectorFormat=1-D array  Unit=N*m  AffineConversion=off
  Product : Product
  Scope : Scope
      settings: ActiveDisplayYMinimum=-3709.91443  ActiveDisplayYMaximum=2185.74477
  Shaft speed : Constant  Value=3600
  Simulink-PS Converter : nesl_utility/Simulink-PS Converter  PhysicalDomain=network_engine_domain  SubClassName=ps_input  LeftPortType=input  RightPortType=output  PseudoPeriodic=off  Frequencies=[]  NoiseDistribution=none  NoiseParameters=[]  Unit=rpm  AffineConversion=off  FilteringAndDerivatives=provide  SimscapeFilterOrder=1  InputFilterTimeConstant=0.001  UdotUserProvided=0
  W to MW : Gain  Gain=1e-6
  R : PMIOPort  Side=Left
  Power : Outport  VectorParamsAs1DForOutWhenUnconnected=off
  tag scope: turbine_power=global
  wires:
  Product/1 -> Convert to W/1
  PS-Simulink Converter1/1 -> Display/1, Scope/1, Product/2
  Shaft speed/1 -> Product/1, Simulink-PS Converter/1
  Convert to W/1 -> W to MW/1
  W to MW/1 -> [turbine_power], Power/1  "turbine_power"
  connections:
  Mechanical Rotational Reference/LConn1 -- Ideal Angular Velocity Source/RConn2
  Ideal Torque Sensor/LConn1 -- R/RConn1
  Ideal Torque Sensor/RConn1 -- Ideal Angular Velocity Source/LConn1
  Simulink-PS Converter/RConn1 -- Ideal Angular Velocity Source/RConn1
  Ideal Torque Sensor/RConn2 -- PS-Simulink Converter1/LConn1

== system SMR_1MW_model/sensor ==
  Subsystem7 : Subsystem
  Conn1 : PMIOPort  Side=Left
  tag scope: post_turbine_press_MPa=global, post_turbine_temp_C=global
  wires:
  Subsystem7/1(pressure) -> [post_turbine_press_MPa]  "post_turbine_press_MPa"
  Subsystem7/2(temperature) -> [post_turbine_temp_C]  "post_turbine_temp_C"
  connections:
  Subsystem7/LConn1 -- Conn1/RConn1

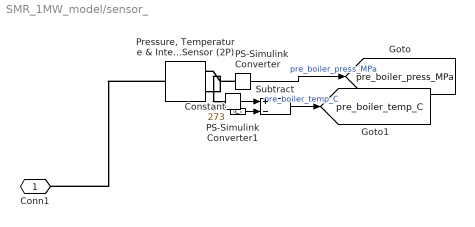
== system SMR_1MW_model/sensor_ ==
  Constant : Constant  Value=273
  PS-Simulink Converter : nesl_utility/PS-Simulink Converter  PhysicalDomain=network_engine_domain  SubClassName=ps_output  LeftPortType=input  RightPortType=output  PseudoPeriodic=off  Frequencies=[]  VectorFormat=inherit  Unit=inherit  AffineConversion=off
  PS-Simulink Converter1 : nesl_utility/PS-Simulink Converter  PhysicalDomain=network_engine_domain  SubClassName=ps_output  LeftPortType=input  RightPortType=output  PseudoPeriodic=off  Frequencies=[]  VectorFormat=inherit  Unit=inherit  AffineConversion=off
  "Pressure, Temperature & Internal Energy Sensor (2P)" : fl_lib/Two-Phase Fluid/Sensors/Pressure, Temperature & Internal Energy Sensor (2P)  reference=foundation.enum.MeasurementReference.absolute  pressure=true  pressure_spec=foundation.enum.PressureMeasementSpec.Absolute  temperature=true  internal_energy=false
      settings: InternalSimscapePortConfiguration="{\"Bottom\":[{\"id\":\"T\",\"label\":\"T\",\"type\":\"output\"}],\"Left\":[{\"id\":\"A\",\"label\":\"A\",\"type\":\"foundation.two_phase_fluid.two_phase_fluid\"}],\"Right\":[{\"id\":\"Pa\",\"label\":\"Pa\",\"type\":\"output\"}],\"Top\":[]}"
  Subtract : Sum  Inputs=+-
  Conn1 : PMIOPort  Side=Left
  tag scope: pre_boiler_press_MPa=global, pre_boiler_temp_C=global
  wires:
  PS-Simulink Converter/1 -> [pre_boiler_press_MPa]  "pre_boiler_press_MPa"
  PS-Simulink Converter1/1 -> Subtract/1
  Constant/1 -> Subtract/2
  Subtract/1 -> [pre_boiler_temp_C]  "pre_boiler_temp_C"
  connections:
  PS-Simulink Converter/LConn1 -- "Pressure, Temperature & Internal Energy Sensor (2P)"/RConn1
  "Pressure, Temperature & Internal Energy Sensor (2P)"/RConn2 -- PS-Simulink Converter1/LConn1
  "Pressure, Temperature & Internal Energy Sensor (2P)"/LConn1 -- Conn1/RConn1

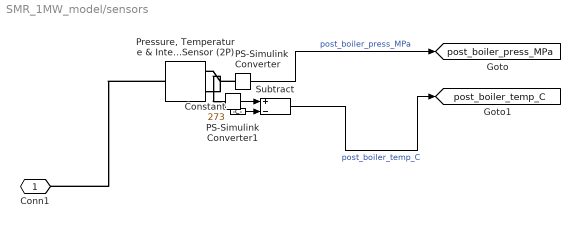
== system SMR_1MW_model/sensors ==
  Constant : Constant  Value=273
  PS-Simulink Converter : nesl_utility/PS-Simulink Converter  PhysicalDomain=network_engine_domain  SubClassName=ps_output  LeftPortType=input  RightPortType=output  PseudoPeriodic=off  Frequencies=[]  VectorFormat=inherit  Unit=inherit  AffineConversion=off
  PS-Simulink Converter1 : nesl_utility/PS-Simulink Converter  PhysicalDomain=network_engine_domain  SubClassName=ps_output  LeftPortType=input  RightPortType=output  PseudoPeriodic=off  Frequencies=[]  VectorFormat=inherit  Unit=inherit  AffineConversion=off
  "Pressure, Temperature & Internal Energy Sensor (2P)" : fl_lib/Two-Phase Fluid/Sensors/Pressure, Temperature & Internal Energy Sensor (2P)  reference=foundation.enum.MeasurementReference.absolute  pressure=true  pressure_spec=foundation.enum.PressureMeasementSpec.Absolute  temperature=true  internal_energy=false
      settings: InternalSimscapePortConfiguration="{\"Bottom\":[{\"id\":\"T\",\"label\":\"T\",\"type\":\"output\"}],\"Left\":[{\"id\":\"A\",\"label\":\"A\",\"type\":\"foundation.two_phase_fluid.two_phase_fluid\"}],\"Right\":[{\"id\":\"Pa\",\"label\":\"Pa\",\"type\":\"output\"}],\"Top\":[]}"
  Subtract : Sum  Inputs=+-
  Conn1 : PMIOPort  Side=Right
  tag scope: post_boiler_press_MPa=global, post_boiler_temp_C=global
  wires:
  PS-Simulink Converter/1 -> [post_boiler_press_MPa]  "post_boiler_press_MPa"
  PS-Simulink Converter1/1 -> Subtract/1
  Constant/1 -> Subtract/2
  Subtract/1 -> [post_boiler_temp_C]  "post_boiler_temp_C"
  connections:
  PS-Simulink Converter/LConn1 -- "Pressure, Temperature & Internal Energy Sensor (2P)"/RConn1
  "Pressure, Temperature & Internal Energy Sensor (2P)"/RConn2 -- PS-Simulink Converter1/LConn1
  "Pressure, Temperature & Internal Energy Sensor (2P)"/LConn1 -- Conn1/RConn1

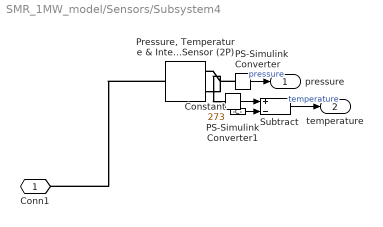
== system SMR_1MW_model/Sensors/Subsystem4 ==
  Constant : Constant  Value=273
  PS-Simulink Converter : nesl_utility/PS-Simulink Converter  PhysicalDomain=network_engine_domain  SubClassName=ps_output  LeftPortType=input  RightPortType=output  PseudoPeriodic=off  Frequencies=[]  VectorFormat=inherit  Unit=inherit  AffineConversion=off
  PS-Simulink Converter1 : nesl_utility/PS-Simulink Converter  PhysicalDomain=network_engine_domain  SubClassName=ps_output  LeftPortType=input  RightPortType=output  PseudoPeriodic=off  Frequencies=[]  VectorFormat=inherit  Unit=inherit  AffineConversion=off
  "Pressure, Temperature & Internal Energy Sensor (2P)" : fl_lib/Two-Phase Fluid/Sensors/Pressure, Temperature & Internal Energy Sensor (2P)  reference=foundation.enum.MeasurementReference.absolute  pressure=true  pressure_spec=foundation.enum.PressureMeasementSpec.Absolute  temperature=true  internal_energy=false
      settings: InternalSimscapePortConfiguration="{\"Bottom\":[{\"id\":\"T\",\"label\":\"T\",\"type\":\"output\"}],\"Left\":[{\"id\":\"A\",\"label\":\"A\",\"type\":\"foundation.two_phase_fluid.two_phase_fluid\"}],\"Right\":[{\"id\":\"Pa\",\"label\":\"Pa\",\"type\":\"output\"}],\"Top\":[]}"
  Subtract : Sum  Inputs=+-
  Conn1 : PMIOPort  Side=Left
  pressure : Outport
  temperature : Outport  Port=2
  wires:
  PS-Simulink Converter/1 -> pressure/1  "pressure"
  PS-Simulink Converter1/1 -> Subtract/1
  Constant/1 -> Subtract/2
  Subtract/1 -> temperature/1  "temperature"
  connections:
  PS-Simulink Converter/LConn1 -- "Pressure, Temperature & Internal Energy Sensor (2P)"/RConn1
  "Pressure, Temperature & Internal Energy Sensor (2P)"/RConn2 -- PS-Simulink Converter1/LConn1
  "Pressure, Temperature & Internal Energy Sensor (2P)"/LConn1 -- Conn1/RConn1

== system SMR_1MW_model/Steam Boiler1/Boiler Heat Flow Sensor ==
  Heat Flow Rate Sensor : fl_lib/Thermal/Thermal Sensors/Heat Flow Rate Sensor
  PS-Simulink Converter : nesl_utility/PS-Simulink Converter  PhysicalDomain=network_engine_domain  SubClassName=ps_output  LeftPortType=input  RightPortType=output  PseudoPeriodic=off  Frequencies=[]  VectorFormat=1-D array  Unit=MW  AffineConversion=off
  A : PMIOPort  Side=Left
  B : PMIOPort  Port=2  Side=Right
  tag scope: Boiler=global
  wires:
  PS-Simulink Converter/1 -> [Boiler]
  connections:
  Heat Flow Rate Sensor/RConn2 -- B/RConn1
  Heat Flow Rate Sensor/LConn1 -- A/RConn1
  Heat Flow Rate Sensor/RConn1 -- PS-Simulink Converter/LConn1

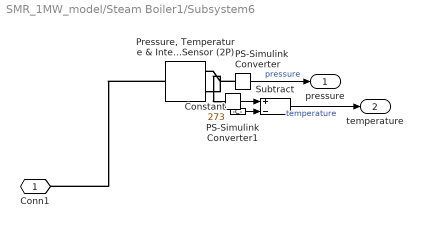
== system SMR_1MW_model/Steam Boiler1/Subsystem6 ==
  Constant : Constant  Value=273
  PS-Simulink Converter : nesl_utility/PS-Simulink Converter  PhysicalDomain=network_engine_domain  SubClassName=ps_output  LeftPortType=input  RightPortType=output  PseudoPeriodic=off  Frequencies=[]  VectorFormat=inherit  Unit=inherit  AffineConversion=off
  PS-Simulink Converter1 : nesl_utility/PS-Simulink Converter  PhysicalDomain=network_engine_domain  SubClassName=ps_output  LeftPortType=input  RightPortType=output  PseudoPeriodic=off  Frequencies=[]  VectorFormat=inherit  Unit=inherit  AffineConversion=off
  "Pressure, Temperature & Internal Energy Sensor (2P)" : fl_lib/Two-Phase Fluid/Sensors/Pressure, Temperature & Internal Energy Sensor (2P)  reference=foundation.enum.MeasurementReference.absolute  pressure=true  pressure_spec=foundation.enum.PressureMeasementSpec.Absolute  temperature=true  internal_energy=false
      settings: InternalSimscapePortConfiguration="{\"Bottom\":[{\"id\":\"T\",\"label\":\"T\",\"type\":\"output\"}],\"Left\":[{\"id\":\"A\",\"label\":\"A\",\"type\":\"foundation.two_phase_fluid.two_phase_fluid\"}],\"Right\":[{\"id\":\"Pa\",\"label\":\"Pa\",\"type\":\"output\"}],\"Top\":[]}"
  Subtract : Sum  Inputs=+-
  Conn1 : PMIOPort  Side=Left
  pressure : Outport
  temperature : Outport  Port=2
  wires:
  PS-Simulink Converter/1 -> pressure/1  "pressure"
  PS-Simulink Converter1/1 -> Subtract/1
  Constant/1 -> Subtract/2
  Subtract/1 -> temperature/1  "temperature"
  connections:
  PS-Simulink Converter/LConn1 -- "Pressure, Temperature & Internal Energy Sensor (2P)"/RConn1
  "Pressure, Temperature & Internal Energy Sensor (2P)"/RConn2 -- PS-Simulink Converter1/LConn1
  "Pressure, Temperature & Internal Energy Sensor (2P)"/LConn1 -- Conn1/RConn1

== system SMR_1MW_model/Steam Boiler1/Superheater Heat Flow Sensor ==
  Heat Flow Rate Sensor : fl_lib/Thermal/Thermal Sensors/Heat Flow Rate Sensor
  PS-Simulink Converter : nesl_utility/PS-Simulink Converter  PhysicalDomain=network_engine_domain  SubClassName=ps_output  LeftPortType=input  RightPortType=output  PseudoPeriodic=off  Frequencies=[]  VectorFormat=1-D array  Unit=MW  AffineConversion=off
  A : PMIOPort  Side=Left
  B : PMIOPort  Port=2  Side=Right
  tag scope: Superheat=global
  wires:
  PS-Simulink Converter/1 -> [Superheat]
  connections:
  Heat Flow Rate Sensor/RConn1 -- PS-Simulink Converter/LConn1
  Heat Flow Rate Sensor/LConn1 -- A/RConn1
  Heat Flow Rate Sensor/RConn2 -- B/RConn1

== system SMR_1MW_model/Steam Boiler1/temp_profile ==
  Add : Sum
  Ramp : simulink/Sources/Ramp  slope=2  start=0  InitialOutput=50
  Ramp1 : simulink/Sources/Ramp  slope=-2  start=T_furnace/2  InitialOutput=0
  Simulink-PS Converter : nesl_utility/Simulink-PS Converter  PhysicalDomain=network_engine_domain  SubClassName=ps_input  LeftPortType=input  RightPortType=output  PseudoPeriodic=off  Frequencies=[]  NoiseDistribution=none  NoiseParameters=[]  Unit=1  AffineConversion=off  FilteringAndDerivatives=provide  SimscapeFilterOrder=1  InputFilterTimeConstant=0.001  UdotUserProvided=0
  output : PMIOPort  Side=Left
  Out1 : Outport
  wires:
  Ramp1/1 -> Add/2
  Ramp/1 -> Add/1
  Add/1 -> Out1/1, Simulink-PS Converter/1
  connections:
  Simulink-PS Converter/RConn1 -- output/RConn1

== system SMR_1MW_model/Steam Condenser1/Condenser Heat Flow Sensor ==
  Heat Flow Rate Sensor : fl_lib/Thermal/Thermal Sensors/Heat Flow Rate Sensor
  A : PMIOPort  Side=Left
  B : PMIOPort  Port=2  Side=Right
  connections:
  Heat Flow Rate Sensor/RConn2 -- B/RConn1
  Heat Flow Rate Sensor/LConn1 -- A/RConn1

== system SMR_1MW_model/sensor/Subsystem7 ==
  Constant : Constant  Value=273
  PS-Simulink Converter : nesl_utility/PS-Simulink Converter  PhysicalDomain=network_engine_domain  SubClassName=ps_output  LeftPortType=input  RightPortType=output  PseudoPeriodic=off  Frequencies=[]  VectorFormat=inherit  Unit=inherit  AffineConversion=off
  PS-Simulink Converter1 : nesl_utility/PS-Simulink Converter  PhysicalDomain=network_engine_domain  SubClassName=ps_output  LeftPortType=input  RightPortType=output  PseudoPeriodic=off  Frequencies=[]  VectorFormat=inherit  Unit=inherit  AffineConversion=off
  "Pressure, Temperature & Internal Energy Sensor (2P)" : fl_lib/Two-Phase Fluid/Sensors/Pressure, Temperature & Internal Energy Sensor (2P)  reference=foundation.enum.MeasurementReference.absolute  pressure=true  pressure_spec=foundation.enum.PressureMeasementSpec.Absolute  temperature=true  internal_energy=false
      settings: InternalSimscapePortConfiguration="{\"Bottom\":[{\"id\":\"T\",\"label\":\"T\",\"type\":\"output\"}],\"Left\":[{\"id\":\"A\",\"label\":\"A\",\"type\":\"foundation.two_phase_fluid.two_phase_fluid\"}],\"Right\":[{\"id\":\"Pa\",\"label\":\"Pa\",\"type\":\"output\"}],\"Top\":[]}"
  Subtract : Sum  Inputs=+-
  Conn1 : PMIOPort  Side=Left
  pressure : Outport
  temperature : Outport  Port=2
  wires:
  PS-Simulink Converter/1 -> pressure/1  "pressure"
  PS-Simulink Converter1/1 -> Subtract/1
  Constant/1 -> Subtract/2
  Subtract/1 -> temperature/1  "temperature"
  connections:
  PS-Simulink Converter/LConn1 -- "Pressure, Temperature & Internal Energy Sensor (2P)"/RConn1
  "Pressure, Temperature & Internal Energy Sensor (2P)"/RConn2 -- PS-Simulink Converter1/LConn1
  "Pressure, Temperature & Internal Energy Sensor (2P)"/LConn1 -- Conn1/RConn1
